simulink model "LoadSense_harness"  (Simulink 7.7)
settings: Solver=FixedStepDiscrete  SolverMode=SingleTasking  StartTime=0.0  StopTime=200  FixedStep=.01  RelTol=1e-3
PostLoadFcn:
  | cd '..';
  | PostLoadFcn;
  | cd 'harness';
InitFcn:
  | if signalbuilder('LoadSense_harness/Signal_Builder','activegroup') == 1
  |   CD_LOADSENSE_FUNCTION.DataType = 'uint8';
  |   CD_LOADSENSE_FUNCTION.Value = 0;
  |   CD_LOADSENSE_REFERENCE.DataType = 'uint8';
  |   CD_LOADSENSE_REFERENCE.Value = 1;
  | elseif signalbuilder('LoadSense_harness/Signal_Builder','activegroup') == 2
  |   CD_LOADSENSE_FUNCTION.DataType = 'uint8';
  |   CD_LOADSENSE_FUNCTION.Value = 255;
  |   CD_LOADSENSE_REFERENCE.DataType = 'uint8';
  |   CD_LOADSENSE_REFERENCE.Value = 1;
  | elseif signalbuilder('LoadSense_harness/Signal_Builder','activegroup') == 3
  |   CD_LOADSENSE_FUNCTION.DataType = 'uint8';
  |   CD_LOADSENSE_FUNCTION.Value = 255;
  |   CD_LOADSENSE_REFERENCE.DataType = 'uint8';
  |   CD_LOADSENSE_REFERENCE.Value = 2;
  | elseif signalbuilder('LoadSense_harness/Signal_Builder','activegroup') == 4
  |   CD_LOADSENSE_FUNCTION.DataType = 'uint8';
  |   CD_LOADSENSE_FUNCTION.Value = 0;
  |   CD_LOADSENSE_REFERENCE.DataType = 'uint8';
  |   CD_LOADSENSE_REFERENCE.Value = 2;
  | end
undefined symbols (not defined in the file): CD_LOADSENSE_DB, CD_LOADSENSE_GAIN, CD_LOADSENSE_OFFSET, CD_LOADSENSE_OORH, CD_LOADSENSE_OORL, CD_LOADSENSE_VOLTS_GAIN, NON_FUNCTIONAL, NORMAL, OORH, OORL, sigbuilder_block, srate, SYS_NORMAL
libraries: simulink x2, MX_Library x1
settings Model: Creator=smindema  LastModifiedBy=zdoll  RecordCoverage=on  CovMetricSettings=dcmw  CovHTMLOptions=-aTS=1 -bRG=1 -bTC=1 -hTR=0 -nFC=0 -scm=1 -bcm=1 -xEv=0  CovCumulativeReport=on
settings MATStruct: SampleTime=0.01  Offset=0  Priority=[1.0]
settings DataIOCC: LimitDataPoints=off  SaveOutput=off  SaveTime=off
settings OptimizationCC: BlockReduction=off  InlineParams=on  ExpressionFolding=off  StateBitsets=on  DataBitsets=on  UseTempVars=on  InitFltsAndDblsToZero=on  NoFixptDivByZeroProtection=on  EfficientFloat2IntCast=on  OptimizeModelRefInitCode=on
settings DebuggingCC: SaveWithParameterizedLinksMsg=none  MultiTaskDSMMsg=warning  MultiTaskCondExecSysMsg=none  IntegerOverflowMsg=none  ModelReferenceCSMismatchMessage=warning
settings HardwareCC: ProdBitPerInt=16  ProdBitPerPointer=16  ProdIntDivRoundTo=Floor  ProdEndianess=BigEndian  ProdWordSize=16  ProdHWDeviceType=Motorola HC12
settings ModelReferenceCC: ModelReferenceNumInstancesAllowed=Single
settings RTWCC: SystemTargetFile=ert.tlc  GenCodeOnly=on  TemplateMakefile=ert_default_tmf  Description=Real-Time Workshop Embedded Coder (no auto configuration)  GenerateReport=on  RetainRTWFile=on  ProcessScript=ert_make_rtw_hook  IncludeHyperlinkInReport=on  LaunchReport=on  IncludeERTFirstTime=on
settings RTWCC: CustomHeaderCode=|
  | #include "cpp_req_defines.h"
  | #include "hw_fin.h"
  | #include "cdata.h"
settings CodeAppCC: IgnoreCustomStorageClasses=off  DefineNamingRule=UpperCase
settings ERTTargetCC: TargetFcnLib=ansi_tfl_tmw.mat  FunctionExecutionProfile=off  MultiwordLength=2048  GenerateSampleERTMain=on  IncludeMdlTerminateFcn=off  SupportAbsoluteTime=off  SupportNonFinite=off  SupportComplex=off  PurelyIntegerCode=on  ERTCustomFileTemplate=gen_rtw_req_defines_h.tlc  GlobalDataDefinition=InSeparateSourceFile  GlobalDataReference=InSeparateHeaderFile  ConvertIfToSwitch=off

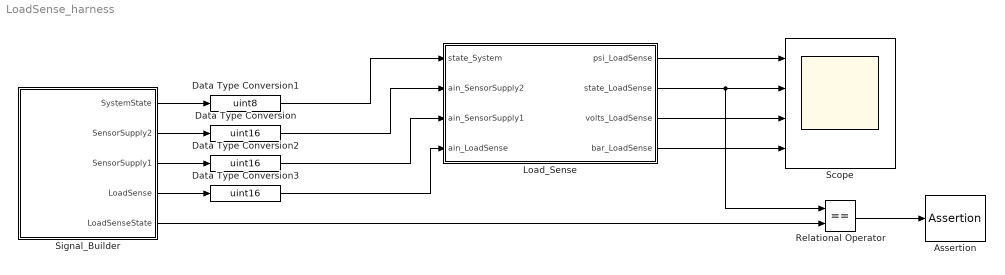
== system LoadSense_harness ==
  Assertion : Assertion  Enabled=on  StopWhenAssertionFail=off
  Data Type Conversion : DataTypeConversion  OutDataTypeStr=uint16  SampleTime=srate
  Data Type Conversion1 : DataTypeConversion  OutDataTypeStr=uint8  SampleTime=srate
  Data Type Conversion2 : DataTypeConversion  OutDataTypeStr=uint16  SampleTime=srate
  Data Type Conversion3 : DataTypeConversion  OutDataTypeStr=uint16  SampleTime=srate
  Load_Sense : Subsystem  TreatAsAtomicUnit=on  SystemSampleTime=srate  RTWFileName=mod_Inputs
      settings: RTWSystemCode=Function  RTWFcnNameOpts=Use subsystem name  RTWFileNameOpts=User specified
  Relational Operator : RelationalOperator  Operator===  OutDataTypeStr=boolean
  Scope : Scope  NumInputPorts=4
      settings: YMin=7.6~-5~-5~-5  YMax=8.4~5~5~5
  Signal_Builder : Subsystem  Tag=STV Subsys  LoadFcn=sigbuilder_block('load');  StartFcn=sigbuilder_block('start');  StopFcn=sigbuilder_block('stop');  ClipboardFcn=sigbuilder_block('clipboard');  mask(Sigbuilder block){}
      mask help: Sigbuilder GUI
      mask init:
      | if ~strcmp(get_param(bdroot(gcbh),'SimulationStatus'),'stopped') tuvar = sigbuilder_block('maskInit'); end
      settings: CopyFcn=sigbuilder_block('copy');  DeleteFcn=sigbuilder_block('delete');  ModelCloseFcn=sigbuilder_block('modelClose');  PreSaveFcn=sigbuilder_block('preSave');  NameChangeFcn=sigbuilder_block('namechange');  OpenFcn=sigbuilder_block('open',[6 28.5 1428 808.5 ]);  CloseFcn=sigbuilder_block('close');
      mask Display: plot(0,0,100,100,[10,10,40,40,10],[80,20,20,80,80],[40,10],[50,50], [40,27,10],[65,72,56],[40,25,25,10],[28,28,43,43]);
  wires:
  Signal_Builder/2(SensorSupply2) -> Data Type Conversion/1
  Relational Operator/1 -> Assertion/1
  Signal_Builder/5(LoadSenseState) -> Relational Operator/2
  Signal_Builder/1(SystemState) -> Data Type Conversion1/1
  Load_Sense/1(psi_LoadSense) -> Scope/1
  Load_Sense/2(state_LoadSense) -> Scope/2, Relational Operator/1
  Load_Sense/3(volts_LoadSense) -> Scope/3
  Load_Sense/4(bar_LoadSense) -> Scope/4
  Signal_Builder/3(SensorSupply1) -> Data Type Conversion2/1
  Data Type Conversion1/1 -> Load_Sense/1(state_System)
  Data Type Conversion/1 -> Load_Sense/2(ain_SensorSupply2)
  Data Type Conversion2/1 -> Load_Sense/3(ain_SensorSupply1)
  Data Type Conversion3/1 -> Load_Sense/4(ain_LoadSense)
  Signal_Builder/4(LoadSense) -> Data Type Conversion3/1

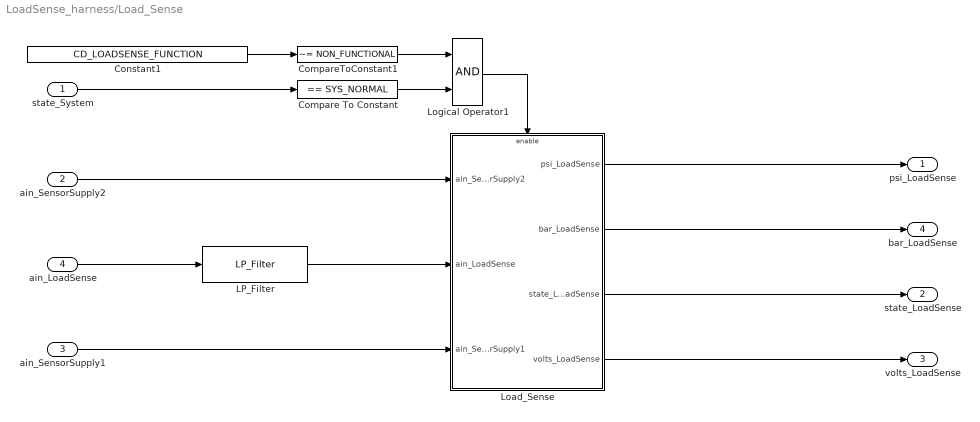
== system LoadSense_harness/Load_Sense ==
  state_System : Inport
  ain_SensorSupply2 : Inport  Port=2
  ain_SensorSupply1 : Inport  Port=3
  ain_LoadSense : Inport  Port=4
  Compare To Constant : simulink/Logic and Bit Operations/Compare To Constant  SystemSampleTime=-1  relop===  const=SYS_NORMAL  LogicOutDataTypeMode=boolean
  CompareToConstant1 : simulink/Logic and Bit Operations/Compare To Constant  SystemSampleTime=-1  relop=~=  const=NON_FUNCTIONAL  LogicOutDataTypeMode=boolean  ZeroCross=off
  Constant1 : Constant  Value=CD_LOADSENSE_FUNCTION
  LP_Filter : MX_Library/LP_Filter  SystemSampleTime=-1  GAIN=CD_LOADSENSE_FILTER_GAIN
  Load_Sense : Subsystem
  Logical Operator1 : Logic  AllPortsSameDT=off  OutDataTypeStr=boolean
  psi_LoadSense : Outport
  state_LoadSense : Outport  Port=2
  volts_LoadSense : Outport  Port=3
  bar_LoadSense : Outport  Port=4
  wires:
  ain_SensorSupply2/1 -> Load_Sense/1(ain_SensorSupply2)
  ain_LoadSense/1 -> LP_Filter/1
  Load_Sense/1(psi_LoadSense) -> psi_LoadSense/1
  Load_Sense/3(state_LoadSense) -> state_LoadSense/1
  ain_SensorSupply1/1 -> Load_Sense/3(ain_SensorSupply1)
  Load_Sense/4(volts_LoadSense) -> volts_LoadSense/1
  state_System/1 -> Compare To Constant/1
  CompareToConstant1/1 -> Logical Operator1/1
  Constant1/1 -> CompareToConstant1/1
  Compare To Constant/1 -> Logical Operator1/2
  Logical Operator1/1 -> Load_Sense/Enable
  Load_Sense/2(bar_LoadSense) -> bar_LoadSense/1
  LP_Filter/1 -> Load_Sense/2(ain_LoadSense)

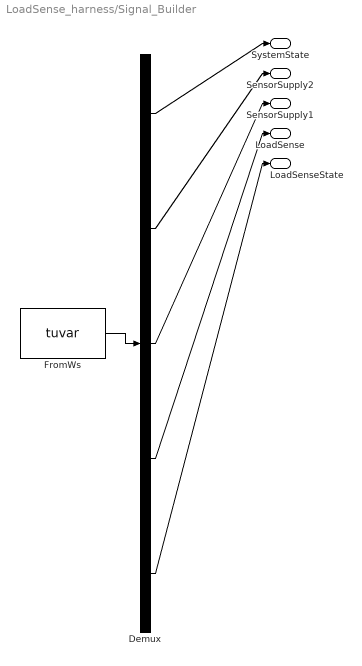
== system LoadSense_harness/Signal_Builder ==
  Demux : Demux  Tag=STV Demux  Outputs=5
  FromWs : FromWorkspace  Tag=STV FromWs  VariableName=tuvar  SampleTime=0  SigBuilderData=DataTag0  VnvData=DataTag1
      SigBuilderData=|
      | common.afterFinalStr = 'Extrapolate'
      | common.sampleTime = 0
      | dataSet(1).timeRange = [0 200]
      | dataSet(1).name = 'Group 1'
      | dataSet(2).timeRange = [0 200]
      | dataSet(2).name = 'Group 2'
      | dataSet(3).timeRange = [0 200]
      | dataSet(3).name = 'Group 3'
      | dataSet(4).timeRange = [0 200]
      | dataSet(4).name = 'Group 4'
      | sbobj.Groups(1).Name = 'Group 1'
      | sbobj.Groups(1).Signals(1).Name = 'SystemState'
      | sbobj.Groups(1).Signals(1).XData = [0 100 100 200]
      | sbobj.Groups(1).Signals(1).YData = [1 1 0 0]
      | sbobj.Groups(1).Signals(2).Name = 'SensorSupply2'
      | sbobj.Groups(1).Signals(2).XData = [0 30 30 60 60 90 90 130 130 160 160 190 190 200]
      | sbobj.Groups(1).Signals(2).YData = [5 5 0 0 12 12 5 5 0 0 12 12 5 5]
      | sbobj.Groups(1).Signals(3).Name = 'SensorSupply1'
      | sbobj.Groups(1).Signals(3).XData = [0 10 10 20 20 30 30 40 40 50 50 60 60 70 70 80 80 90 90 110 110 120 120 130 130 140 140 150 150 160 160 170 170 180 180 190 190 200]
      | sbobj.Groups(1).Signals(3).YData = [8 8 0 0 12 12 8 8 0 0 12 12 8 8 0 0 12 12 8 8 0 0 12 12 8 8 0 0 12 12 8 8 0 0 12 12 8 8]
      | sbobj.Groups(1).Signals(4).Name = 'LoadSense'
      | sbobj.Groups(1).Signals(4).XData = [0 0.5 0.5 1 1 2.5 2.5 4 4 4.5 4.5 5 5 6.5 6.5 10 10 10.5 10.5 11 11 12.5 12.5 14 14 14.5 14.5 15 15 16.5 16.5 20 20 20.5 20.5 21 21 22.5 22.5 24 24 24.5 24.5 25 25 26.5 26.5 30 30 30.5 30.5 31 31 32.5 32.5 34 34 34.5 34.5 35 35 36.5 36.5 40 40 40.5 40.5 41 41 42.5 42.5 44 44 44.5 44.5 45 45 46.5 46.5 50 50 50.5 50.5 51 51 52.5 52.5 54 54 54.5 54.5 55 55 56.5 56.5 60 60 60.5 60.5 61 61 62.5 62.5 64 64 64.5 64.5 65 65 66.5 66.5 70 70 70.5 70.5 71 71 72.5 72.5 74 74 74.5 74.5 75 75 76.5 76.5 80 80 80.5 80.5 81 81 82.5 82.5 84 84 84.5 84.5 85 85 86.5 86.5 90 90 90.5 90.5 91 91 92.5 92.5 94 94 94.5 94.5 95 95 96.5 96.5 100 100 100.5 100.5 101 101 102.5 102.5 104 104 104.5 104.5 105 105 106.5 106.5 110 110 110.5 110.5 111 111 112.5 112.5 114 114 114.5 114.5 115 115 116.5 116.5 120 120 120.5 120.5 121 121 122.5 122.5 124 124 124.5 124.5 125 125 126.5 126.5 130 130 130.5 130.5 131 131 132.5 132.5 134 134 134.5 134.5 135 135 136.5 136.5 140 140 140.5 140.5 141 141 142.5 142.5 144 144 144.5 144.5 145 145 146.5 146.5 150 150 150.5 150.5 151 151 152.5 152.5 154 154 154.5 154.5 155 155 156.5 156.5 160 160 160.5 160.5 161 161 162.5 162.5 164 164 164.5 164.5 165 165 166.5 166.5 170 170 170.5 170.5 171 171 172.5 172.5 174 174 174.5 174.5 175 175 176.5 176.5 180 180 180.5 180.5 181 181 182.5 182.5 184 184 184.5 184.5 185 185 186.5 186.5 190 190 190.5 190.5 191 191 192.5 192.5 194 194 194.5 194.5 195 195 196.5 196.5 200]
      | sbobj.Groups(1).Signals(4).YData = [0 0 4 4 0 0 4 4 12 12 5 5 12 12 0 12 0 0 4 4 0 0 4 4 12 12 5 5 12 12 0 12 0 0 4 4 0 0 4 4 12 12 5 5 12 12 0 12 0 0 4 4 0 0 4 4 12 12 5 5 12 12 0 12 0 0 4 4 0 0 4 4 12 12 5 5 12 12 0 12 0 0 4 4 0 0 4 4 12 12 5 5 12 12 0 12 0 0 4 4 0 0 4 4 12 12 5 5 12 12 0 12 0 0 4 4 0 0 4 4 12 12 5 5 12 12 0 12 0 0 4 4 0 0 4 4 12 12 5 5 12 12 0 12 0 0 4 4 0 0 4 4 12 12 5 5 12 12 0 12 0 0 4 4 0 0 4 4 12 12 5 5 12 12 0 12 0 0 4 4 0 0 4 4 12 12 5 5 12 12 0 12 0 0 4 4 0 0 4 4 12 12 5 5 12 12 0 12 0 0 4 4 0 0 4 4 12 12 5 5 12 12 0 12 0 0 4 4 0 0 4 4 12 12 5 5 12 12 0 12 0 0 4 4 0 0 4 4 12 12 5 5 12 12 0 12 0 0 4 4 0 0 4 4 12 12 5 5 12 12 0 12 0 0 4 4 0 0 4 4 12 12 5 5 12 12 0 12 0 0 4 4 0 0 4 4 12 12 5 5 12 12 0 12 0 0 4 4 0 0 4 4 12 12 5 5 12 12 0 12]
      | sbobj.Groups(1).Signals(5).Name = 'LoadSenseState'
      | sbobj.Groups(1).Signals(5).XData = [0 2.16 2.17 3.49 3.5 4.99 5 7.8 7.81 9.03 9.04 12.16 12.17 13.49 13.5 14.99 15 17.8 17.81 19.03 19.04 22.16 22.17 23.5 23.5 25 25 27.8 27.81 29.03 29.04 62.11 62.12 63.5 63.51 66.14 66.15 67.86 67.87 72.11 72.12 73.5 73.51 76.14 76.15 77.86 77.87 82.11 82.12 83.5 83.51 86.14 86.15 87.86 87.87 92.16 92.17 93.49 93.5 94.99 95 97.8 97.81 99.03 99.04 100 100 200]
      | sbobj.Groups(1).Signals(5).YData = [8 8 22 22 8 8 21 21 8 8 21 21 22 22 8 8 21 21 8 8 21 21 22 22 8 8 21 21 8 8 21 21 22 22 8 8 21 21 8 8 22 22 8 8 21 21 8 8 22 22 8 8 21 21 8 8 22 22 8 8 21 21 8 8 21 21 8 8]
      | sbobj.Groups(1).TimeRange = [0 200]
      | sbobj.Groups(2).Name = 'Group 2'
      | sbobj.Groups(2).Signals(1).Name = 'SystemState'
      | sbobj.Groups(2).Signals(1).XData = [0 100 100 200]
      | sbobj.Groups(2).Signals(1).YData = [1 1 0 0]
      | sbobj.Groups(2).Signals(2).Name = 'SensorSupply2'
      | sbobj.Groups(2).Signals(2).XData = [0 30 30 60 60 90 90 130 130 160 160 190 190 200]
      | sbobj.Groups(2).Signals(2).YData = [5 5 0 0 12 12 5 5 0 0 12 12 5 5]
      | sbobj.Groups(2).Signals(3).Name = 'SensorSupply1'
      | sbobj.Groups(2).Signals(3).XData = [0 10 10 20 20 30 30 40 40 50 50 60 60 70 70 80 80 90 90 110 110 120 120 130 130 140 140 150 150 160 160 170 170 180 180 190 190 200]
      | sbobj.Groups(2).Signals(3).YData = [8 8 0 0 12 12 8 8 0 0 12 12 8 8 0 0 12 12 8 8 0 0 12 12 8 8 0 0 12 12 8 8 0 0 12 12 8 8]
      | sbobj.Groups(2).Signals(4).Name = 'LoadSense'
      | sbobj.Groups(2).Signals(4).XData = [0 0.5 0.5 1 1 2.5 2.5 4 4 4.5 4.5 5 5 6.5 6.5 10 10 10.5 10.5 11 11 12.5 12.5 14 14 14.5 14.5 15 15 16.5 16.5 20 20 20.5 20.5 21 21 22.5 22.5 24 24 24.5 24.5 25 25 26.5 26.5 30 30 30.5 30.5 31 31 32.5 32.5 34 34 34.5 34.5 35 35 36.5 36.5 40 40 40.5 40.5 41 41 42.5 42.5 44 44 44.5 44.5 45 45 46.5 46.5 50 50 50.5 50.5 51 51 52.5 52.5 54 54 54.5 54.5 55 55 56.5 56.5 60 60 60.5 60.5 61 61 62.5 62.5 64 64 64.5 64.5 65 65 66.5 66.5 70 70 70.5 70.5 71 71 72.5 72.5 74 74 74.5 74.5 75 75 76.5 76.5 80 80 80.5 80.5 81 81 82.5 82.5 84 84 84.5 84.5 85 85 86.5 86.5 90 90 90.5 90.5 91 91 92.5 92.5 94 94 94.5 94.5 95 95 96.5 96.5 100 100 100.5 100.5 101 101 102.5 102.5 104 104 104.5 104.5 105 105 106.5 106.5 110 110 110.5 110.5 111 111 112.5 112.5 114 114 114.5 114.5 115 115 116.5 116.5 120 120 120.5 120.5 121 121 122.5 122.5 124 124 124.5 124.5 125 125 126.5 126.5 130 130 130.5 130.5 131 131 132.5 132.5 134 134 134.5 134.5 135 135 136.5 136.5 140 140 140.5 140.5 141 141 142.5 142.5 144 144 144.5 144.5 145 145 146.5 146.5 150 150 150.5 150.5 151 151 152.5 152.5 154 154 154.5 154.5 155 155 156.5 156.5 160 160 160.5 160.5 161 161 162.5 162.5 164 164 164.5 164.5 165 165 166.5 166.5 170 170 170.5 170.5 171 171 172.5 172.5 174 174 174.5 174.5 175 175 176.5 176.5 180 180 180.5 180.5 181 181 182.5 182.5 184 184 184.5 184.5 185 185 186.5 186.5 190 190 190.5 190.5 191 191 192.5 192.5 194 194 194.5 194.5 195 195 196.5 196.5 200]
      | sbobj.Groups(2).Signals(4).YData = [0 0 4 4 0 0 4 4 12 12 5 5 12 12 0 12 0 0 4 4 0 0 4 4 12 12 5 5 12 12 0 12 0 0 4 4 0 0 4 4 12 12 5 5 12 12 0 12 0 0 4 4 0 0 4 4 12 12 5 5 12 12 0 12 0 0 4 4 0 0 4 4 12 12 5 5 12 12 0 12 0 0 4 4 0 0 4 4 12 12 5 5 12 12 0 12 0 0 4 4 0 0 4 4 12 12 5 5 12 12 0 12 0 0 4 4 0 0 4 4 12 12 5 5 12 12 0 12 0 0 4 4 0 0 4 4 12 12 5 5 12 12 0 12 0 0 4 4 0 0 4 4 12 12 5 5 12 12 0 12 0 0 4 4 0 0 4 4 12 12 5 5 12 12 0 12 0 0 4 4 0 0 4 4 12 12 5 5 12 12 0 12 0 0 4 4 0 0 4 4 12 12 5 5 12 12 0 12 0 0 4 4 0 0 4 4 12 12 5 5 12 12 0 12 0 0 4 4 0 0 4 4 12 12 5 5 12 12 0 12 0 0 4 4 0 0 4 4 12 12 5 5 12 12 0 12 0 0 4 4 0 0 4 4 12 12 5 5 12 12 0 12 0 0 4 4 0 0 4 4 12 12 5 5 12 12 0 12 0 0 4 4 0 0 4 4 12 12 5 5 12 12 0 12 0 0 4 4 0 0 4 4 12 12 5 5 12 12 0 12]
      | sbobj.Groups(2).Signals(5).Name = 'LoadSenseState'
      | sbobj.Groups(2).Signals(5).XData = [0 6.8 12.6 200]
      | sbobj.Groups(2).Signals(5).YData = [8 8 8 8]
      | sbobj.Groups(2).TimeRange = [0 200]
      | sbobj.Groups(3).Name = 'Group 3'
      | sbobj.Groups(3).Signals(1).Name = 'SystemState'
      | sbobj.Groups(3).Signals(1).XData = [0 100 100 200]
      | sbobj.Groups(3).Signals(1).YData = [1 1 0 0]
      | sbobj.Groups(3).Signals(2).Name = 'SensorSupply2'
      | sbobj.Groups(3).Signals(2).XData = [0 30 30 60 60 90 90 130 130 160 160 190 190 200]
      | sbobj.Groups(3).Signals(2).YData = [5 5 0 0 12 12 5 5 0 0 12 12 5 5]
      | sbobj.Groups(3).Signals(3).Name = 'SensorSupply1'
      | sbobj.Groups(3).Signals(3).XData = [0 10 10 20 20 30 30 40 40 50 50 60 60 70 70 80 80 90 90 110 110 120 120 130 130 140 140 150 150 160 160 170 170 180 180 190 190 200]
      | sbobj.Groups(3).Signals(3).YData = [8 8 0 0 12 12 8 8 0 0 12 12 8 8 0 0 12 12 8 8 0 0 12 12 8 8 0 0 12 12 8 8 0 0 12 12 8 8]
      | sbobj.Groups(3).Signals(4).Name = 'LoadSense'
      | sbobj.Groups(3).Signals(4).XData = [0 0.5 0.5 1 1 2.5 2.5 4 4 4.5 4.5 5 5 6.5 6.5 10 10 10.5 10.5 11 11 12.5 12.5 14 14 14.5 14.5 15 15 16.5 16.5 20 20 20.5 20.5 21 21 22.5 22.5 24 24 24.5 24.5 25 25 26.5 26.5 30 30 30.5 30.5 31 31 32.5 32.5 34 34 34.5 34.5 35 35 36.5 36.5 40 40 40.5 40.5 41 41 42.5 42.5 44 44 44.5 44.5 45 45 46.5 46.5 50 50 50.5 50.5 51 51 52.5 52.5 54 54 54.5 54.5 55 55 56.5 56.5 60 60 60.5 60.5 61 61 62.5 62.5 64 64 64.5 64.5 65 65 66.5 66.5 70 70 70.5 70.5 71 71 72.5 72.5 74 74 74.5 74.5 75 75 76.5 76.5 80 80 80.5 80.5 81 81 82.5 82.5 84 84 84.5 84.5 85 85 86.5 86.5 90 90 90.5 90.5 91 91 92.5 92.5 94 94 94.5 94.5 95 95 96.5 96.5 100 100 100.5 100.5 101 101 102.5 102.5 104 104 104.5 104.5 105 105 106.5 106.5 110 110 110.5 110.5 111 111 112.5 112.5 114 114 114.5 114.5 115 115 116.5 116.5 120 120 120.5 120.5 121 121 122.5 122.5 124 124 124.5 124.5 125 125 126.5 126.5 130 130 130.5 130.5 131 131 132.5 132.5 134 134 134.5 134.5 135 135 136.5 136.5 140 140 140.5 140.5 141 141 142.5 142.5 144 144 144.5 144.5 145 145 146.5 146.5 150 150 150.5 150.5 151 151 152.5 152.5 154 154 154.5 154.5 155 155 156.5 156.5 160 160 160.5 160.5 161 161 162.5 162.5 164 164 164.5 164.5 165 165 166.5 166.5 170 170 170.5 170.5 171 171 172.5 172.5 174 174 174.5 174.5 175 175 176.5 176.5 180 180 180.5 180.5 181 181 182.5 182.5 184 184 184.5 184.5 185 185 186.5 186.5 190 190 190.5 190.5 191 191 192.5 192.5 194 194 194.5 194.5 195 195 196.5 196.5 200]
      | sbobj.Groups(3).Signals(4).YData = [0 0 4 4 0 0 4 4 12 12 5 5 12 12 0 12 0 0 4 4 0 0 4 4 12 12 5 5 12 12 0 12 0 0 4 4 0 0 4 4 12 12 5 5 12 12 0 12 0 0 4 4 0 0 4 4 12 12 5 5 12 12 0 12 0 0 4 4 0 0 4 4 12 12 5 5 12 12 0 12 0 0 4 4 0 0 4 4 12 12 5 5 12 12 0 12 0 0 4 4 0 0 4 4 12 12 5 5 12 12 0 12 0 0 4 4 0 0 4 4 12 12 5 5 12 12 0 12 0 0 4 4 0 0 4 4 12 12 5 5 12 12 0 12 0 0 4 4 0 0 4 4 12 12 5 5 12 12 0 12 0 0 4 4 0 0 4 4 12 12 5 5 12 12 0 12 0 0 4 4 0 0 4 4 12 12 5 5 12 12 0 12 0 0 4 4 0 0 4 4 12 12 5 5 12 12 0 12 0 0 4 4 0 0 4 4 12 12 5 5 12 12 0 12 0 0 4 4 0 0 4 4 12 12 5 5 12 12 0 12 0 0 4 4 0 0 4 4 12 12 5 5 12 12 0 12 0 0 4 4 0 0 4 4 12 12 5 5 12 12 0 12 0 0 4 4 0 0 4 4 12 12 5 5 12 12 0 12 0 0 4 4 0 0 4 4 12 12 5 5 12 12 0 12 0 0 4 4 0 0 4 4 12 12 5 5 12 12 0 12]
      | sbobj.Groups(3).Signals(5).Name = 'LoadSenseState'
      | sbobj.Groups(3).Signals(5).XData = [0 6.8 12.6 200]
      | sbobj.Groups(3).Signals(5).YData = [8 8 8 8]
      | sbobj.Groups(3).TimeRange = [0 200]
      | sbobj.Groups(4).Name = 'Group 4'
      | sbobj.Groups(4).Signals(1).Name = 'SystemState'
      | sbobj.Groups(4).Signals(1).XData = [0 100 100 200]
      | sbobj.Groups(4).Signals(1).YData = [1 1 0 0]
      | sbobj.Groups(4).Signals(2).Name = 'SensorSupply2'
      | sbobj.Groups(4).Signals(2).XData = [0 30 30 60 60 90 90 130 130 160 160 190 190 200]
      | sbobj.Groups(4).Signals(2).YData = [5 5 0 0 12 12 5 5 0 0 12 12 5 5]
      | sbobj.Groups(4).Signals(3).Name = 'SensorSupply1'
      | sbobj.Groups(4).Signals(3).XData = [0 10 10 20 20 30 30 40 40 50 50 60 60 70 70 80 80 90 90 110 110 120 120 130 130 140 140 150 150 160 160 170 170 180 180 190 190 200]
      | sbobj.Groups(4).Signals(3).YData = [8 8 0 0 12 12 8 8 0 0 12 12 8 8 0 0 12 12 8 8 0 0 12 12 8 8 0 0 12 12 8 8 0 0 12 12 8 8]
      | sbobj.Groups(4).Signals(4).Name = 'LoadSense'
      | sbobj.Groups(4).Signals(4).XData = [0 0.5 0.5 1 1 2.5 2.5 4 4 4.5 4.5 5 5 6.5 6.5 10 10 10.5 10.5 11 11 12.5 12.5 14 14 14.5 14.5 15 15 16.5 16.5 20 20 20.5 20.5 21 21 22.5 22.5 24 24 24.5 24.5 25 25 26.5 26.5 30 30 30.5 30.5 31 31 32.5 32.5 34 34 34.5 34.5 35 35 36.5 36.5 40 40 40.5 40.5 41 41 42.5 42.5 44 44 44.5 44.5 45 45 46.5 46.5 50 50 50.5 50.5 51 51 52.5 52.5 54 54 54.5 54.5 55 55 56.5 56.5 60 60 60.5 60.5 61 61 62.5 62.5 64 64 64.5 64.5 65 65 66.5 66.5 70 70 70.5 70.5 71 71 72.5 72.5 74 74 74.5 74.5 75 75 76.5 76.5 80 80 80.5 80.5 81 81 82.5 82.5 84 84 84.5 84.5 85 85 86.5 86.5 90 90 90.5 90.5 91 91 92.5 92.5 94 94 94.5 94.5 95 95 96.5 96.5 100 100 100.5 100.5 101 101 102.5 102.5 104 104 104.5 104.5 105 105 106.5 106.5 110 110 110.5 110.5 111 111 112.5 112.5 114 114 114.5 114.5 115 115 116.5 116.5 120 120 120.5 120.5 121 121 122.5 122.5 124 124 124.5 124.5 125 125 126.5 126.5 130 130 130.5 130.5 131 131 132.5 132.5 134 134 134.5 134.5 135 135 136.5 136.5 140 140 140.5 140.5 141 141 142.5 142.5 144 144 144.5 144.5 145 145 146.5 146.5 150 150 150.5 150.5 151 151 152.5 152.5 154 154 154.5 154.5 155 155 156.5 156.5 160 160 160.5 160.5 161 161 162.5 162.5 164 164 164.5 164.5 165 165 166.5 166.5 170 170 170.5 170.5 171 171 172.5 172.5 174 174 174.5 174.5 175 175 176.5 176.5 180 180 180.5 180.5 181 181 182.5 182.5 184 184 184.5 184.5 185 185 186.5 186.5 190 190 190.5 190.5 191 191 192.5 192.5 194 194 194.5 194.5 195 195 196.5 196.5 200]
      | sbobj.Groups(4).Signals(4).YData = [0 0 4 4 0 0 4 4 12 12 5 5 12 12 0 12 0 0 4 4 0 0 4 4 12 12 5 5 12 12 0 12 0 0 4 4 0 0 4 4 12 12 5 5 12 12 0 12 0 0 4 4 0 0 4 4 12 12 5 5 12 12 0 12 0 0 4 4 0 0 4 4 12 12 5 5 12 12 0 12 0 0 4 4 0 0 4 4 12 12 5 5 12 12 0 12 0 0 4 4 0 0 4 4 12 12 5 5 12 12 0 12 0 0 4 4 0 0 4 4 12 12 5 5 12 12 0 12 0 0 4 4 0 0 4 4 12 12 5 5 12 12 0 12 0 0 4 4 0 0 4 4 12 12 5 5 12 12 0 12 0 0 4 4 0 0 4 4 12 12 5 5 12 12 0 12 0 0 4 4 0 0 4 4 12 12 5 5 12 12 0 12 0 0 4 4 0 0 4 4 12 12 5 5 12 12 0 12 0 0 4 4 0 0 4 4 12 12 5 5 12 12 0 12 0 0 4 4 0 0 4 4 12 12 5 5 12 12 0 12 0 0 4 4 0 0 4 4 12 12 5 5 12 12 0 12 0 0 4 4 0 0 4 4 12 12 5 5 12 12 0 12 0 0 4 4 0 0 4 4 12 12 5 5 12 12 0 12 0 0 4 4 0 0 4 4 12 12 5 5 12 12 0 12 0 0 4 4 0 0 4 4 12 12 5 5 12 12 0 12]
      | sbobj.Groups(4).Signals(5).Name = 'LoadSenseState'
      | sbobj.Groups(4).Signals(5).XData = [0 2.14 2.15 3.49 3.5 6.03 6.03 7.82 7.83 9.88 9.88 22.11 22.12 23.5 23.51 26.14 26.15 27.86 27.87 32.14 32.15 33.49 33.5 36.02 36.03 37.82 37.83 39.87 39.88 52.11 52.12 53.5 53.51 56.14 56.15 57.86 57.87 62.14 62.15 63.49 63.5 66.02 66.03 67.83 67.83 69.87 69.88 82.11 82.12 83.5 83.51 86.14 86.15 87.86 87.87 92.14 92.15 93.49 93.5 96.02 96.03 97.83 97.83 99.87 99.88 100 100 200]
      | sbobj.Groups(4).Signals(5).YData = [8 8 22 22 8 8 21 21 8 8 21 21 22 22 8 8 21 21 8 8 22 22 8 8 21 21 8 8 21 21 22 22 8 8 21 21 8 8 22 22 8 8 21 21 8 8 21 21 22 22 8 8 21 21 8 8 22 22 8 8 21 21 8 8 21 21 8 8]
      | sbobj.Groups(4).TimeRange = [0 200]
  SystemState : Outport  Tag=STV Outport
  SensorSupply2 : Outport  Tag=STV Outport  Port=2
  SensorSupply1 : Outport  Tag=STV Outport  Port=3
  LoadSense : Outport  Tag=STV Outport  Port=4
  LoadSenseState : Outport  Tag=STV Outport  Port=5
  wires:
  FromWs/1 -> Demux/1
  Demux/1 -> SystemState/1
  Demux/2 -> SensorSupply2/1
  Demux/3 -> SensorSupply1/1
  Demux/4 -> LoadSense/1
  Demux/5 -> LoadSenseState/1

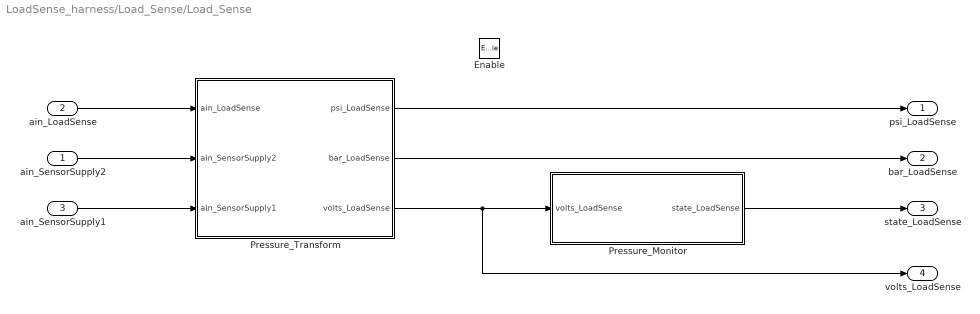
== system LoadSense_harness/Load_Sense/Load_Sense ==
  ain_SensorSupply2 : Inport
  ain_LoadSense : Inport  Port=2
  ain_SensorSupply1 : Inport  Port=3
  Enable : EnablePort  StatesWhenEnabling=reset
  Pressure_Monitor : Stateflow chart  RequirementInfo={} %GIDa_315e9fa6_e0dd_4ab8_9620_290a06eaf03d  TreatAsAtomicUnit=on
  Pressure_Transform : Subsystem
  psi_LoadSense : Outport  OutputWhenDisabled=reset  InitialOutput=[0]
  bar_LoadSense : Outport  Port=2  OutputWhenDisabled=reset  InitialOutput=[0]
  state_LoadSense : Outport  Port=3  OutputWhenDisabled=reset  InitialOutput=[8]
  volts_LoadSense : Outport  Port=4  OutputWhenDisabled=reset  InitialOutput=[0]
  wires:
  Pressure_Transform/3(volts_LoadSense) -> Pressure_Monitor/1(volts_LoadSense), volts_LoadSense/1
  Pressure_Transform/1(psi_LoadSense) -> psi_LoadSense/1
  Pressure_Monitor/1(state_LoadSense) -> state_LoadSense/1
  ain_LoadSense/1 -> Pressure_Transform/1(ain_LoadSense)
  ain_SensorSupply2/1 -> Pressure_Transform/2(ain_SensorSupply2)
  ain_SensorSupply1/1 -> Pressure_Transform/3(ain_SensorSupply1)
  Pressure_Transform/2(bar_LoadSense) -> bar_LoadSense/1

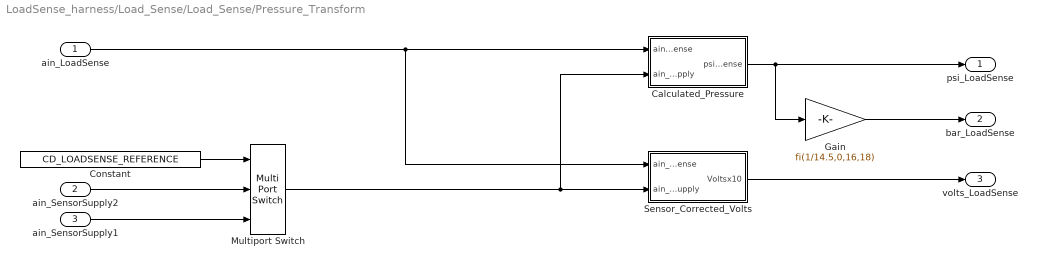
== system LoadSense_harness/Load_Sense/Load_Sense/Pressure_Transform ==
  ain_LoadSense : Inport
  ain_SensorSupply2 : Inport  Port=2
  ain_SensorSupply1 : Inport  Port=3
  Calculated_Pressure : Subsystem  RequirementInfo={} %GIDa_5f6cff1e_8808_4cda_8d6d_a04e247d5c20
  Constant : Constant  RequirementInfo={} %GIDa_1fbd377e_ee87_46ea_8419_8a173a96b5fc  Value=CD_LOADSENSE_REFERENCE  OutDataTypeStr=uint8
  Gain : Gain  Gain=fi(1/14.5,0,16,18)  ParamDataTypeStr=fixdt(0,16,18)  OutDataTypeStr=fixdt(0,16,8)
      settings: AttributesFormatString=Gain = %<Gain>
  Multiport Switch : MultiPortSwitch  Inputs=2  zeroidx=off  InputSameDT=on
  Sensor_Corrected_Volts : Subsystem  RequirementInfo={} %GIDa_801eeb47_ed14_4091_9f9a_39536eca8a32
  psi_LoadSense : Outport
  bar_LoadSense : Outport  Port=2
  volts_LoadSense : Outport  Port=3
  wires:
  Calculated_Pressure/1(psi_Loadsense) -> psi_LoadSense/1, Gain/1
  ain_LoadSense/1 -> Sensor_Corrected_Volts/1(ain_LoadSense), Calculated_Pressure/1(ain_LoadSense)
  Sensor_Corrected_Volts/1(Voltsx10) -> volts_LoadSense/1
  Constant/1 -> Multiport Switch/1
  ain_SensorSupply2/1 -> Multiport Switch/2
  ain_SensorSupply1/1 -> Multiport Switch/3
  Multiport Switch/1 -> Sensor_Corrected_Volts/2(ain_SensorSupply), Calculated_Pressure/2(ain_SensorSupply)
  Gain/1 -> bar_LoadSense/1

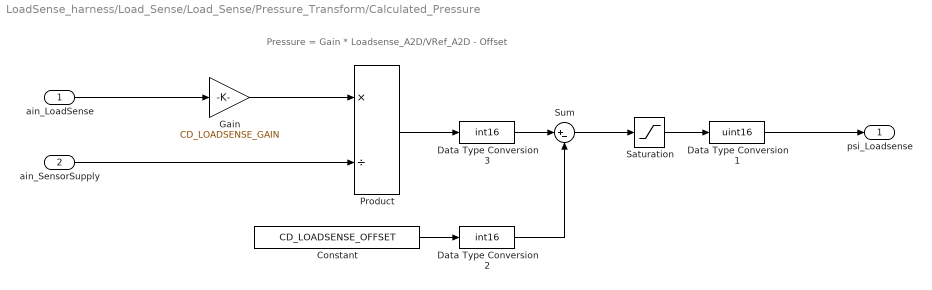
== system LoadSense_harness/Load_Sense/Load_Sense/Pressure_Transform/Calculated_Pressure ==
  note: Pressure = Gain * Loadsense_A2D/VRef_A2D - Offset
  ain_LoadSense : Inport
  ain_SensorSupply : Inport  Port=2
  Constant : Constant  Value=CD_LOADSENSE_OFFSET  OutDataTypeStr=uint16
  Data Type Conversion1 : DataTypeConversion  OutDataTypeStr=uint16
  Data Type Conversion2 : DataTypeConversion  OutDataTypeStr=int16
  Data Type Conversion3 : DataTypeConversion  OutDataTypeStr=int16  SaturateOnIntegerOverflow=on
  Gain : Gain  Gain=CD_LOADSENSE_GAIN  ParamDataTypeStr=uint16  OutMin=0  OutMax=1024*8000  OutDataTypeStr=fixdt(0,32,9)
      settings: AttributesFormatString=Gain = %<Gain>
  Product : Product  Inputs=*/  LockScale=on
  Saturation : Saturate  UpperLimit=8000  LowerLimit=0
      settings: AttributesFormatString=Upper Limit = %<UpperLimit>\nLower Limit = %<LowerLimit>
  Sum : Sum  Inputs=|+-  OutDataTypeStr=int16
  psi_Loadsense : Outport
  wires:
  Saturation/1 -> Data Type Conversion1/1
  ain_LoadSense/1 -> Gain/1
  Gain/1 -> Product/1
  ain_SensorSupply/1 -> Product/2
  Product/1 -> Data Type Conversion3/1
  Constant/1 -> Data Type Conversion2/1
  Sum/1 -> Saturation/1
  Data Type Conversion1/1 -> psi_Loadsense/1
  Data Type Conversion2/1 -> Sum/2
  Data Type Conversion3/1 -> Sum/1

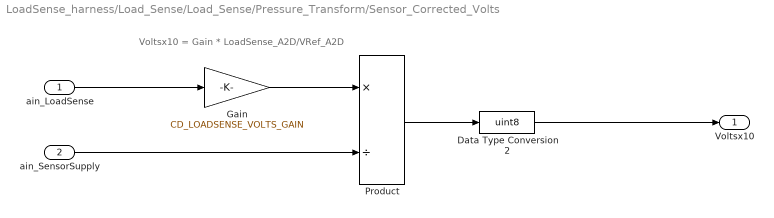
== system LoadSense_harness/Load_Sense/Load_Sense/Pressure_Transform/Sensor_Corrected_Volts ==
  note: Voltsx10 = Gain * LoadSense_A2D/VRef_A2D
  ain_LoadSense : Inport
  ain_SensorSupply : Inport  Port=2
  Data Type Conversion2 : DataTypeConversion  OutDataTypeStr=uint8  SaturateOnIntegerOverflow=on
  Gain : Gain  Gain=CD_LOADSENSE_VOLTS_GAIN  ParamDataTypeStr=fixdt(0,16,9)  OutMax=1024*100  OutDataTypeStr=fixdt(0,32,15)
      settings: AttributesFormatString=Gain = %<Gain>
  Product : Product  Inputs=*/  LockScale=on
  Voltsx10 : Outport
  wires:
  ain_LoadSense/1 -> Gain/1
  Gain/1 -> Product/1
  ain_SensorSupply/1 -> Product/2
  Product/1 -> Data Type Conversion2/1
  Data Type Conversion2/1 -> Voltsx10/1

== stateflow chart Load_Sense/Load_Sense/Pressure_Monitor ==
  state Normal
    state Normal_DB
    state Normal
      en:
      state_LoadSense = NORMAL;
    Normal_DB -> Normal.Normal : [after(CD_LOADSENSE_DB,tick) ||...
        |  state_LoadSense == NORMAL]
    (default) -> Normal_DB
  state OORL_DB
  state OORL
    state_LoadSense = OORL;
  state OORH_DB
  state OORH
    state_LoadSense = OORH;
  state Init
    en:
    state_LoadSense = NORMAL;
  OORH -> Normal : [volts_LoadSense <= CD_LOADSENSE_OORH]
  OORL_DB -> OORL [order 1] : [after(CD_LOADSENSE_DB ,tick)]
  Normal -> OORL_DB [order 1] : [volts_LoadSense < CD_LOADSENSE_OORL]
  OORL_DB -> Normal [order 2] : [volts_LoadSense >= CD_LOADSENSE_OORL]
  OORH_DB -> OORH [order 1] : [after(CD_LOADSENSE_DB ,tick)]
  Normal -> OORH_DB [order 2] : [volts_LoadSense > CD_LOADSENSE_OORH]
  OORH_DB -> Normal [order 2] : [volts_LoadSense <= CD_LOADSENSE_OORH]
  OORL -> Normal : [volts_LoadSense >= CD_LOADSENSE_OORL]
  (default) -> Init
  Init -> Normal
  data: volts_LoadSense input uint8; state_LoadSense output uint8; CD_LOADSENSE_OORH parameter uint8; CD_LOADSENSE_OORL parameter uint8; CD_LOADSENSE_DB parameter uint8; NORMAL parameter uint8; OORH parameter uint8; OORL parameter uint8
